simulink model "ExRobotAndEnvironmentControllerContPI"  (Simulink 8.9)
settings: Solver=ode45  StartTime=0.0  StopTime=1000  FixedStep=.01  RelTol=1e-3  EnableMultiTasking=on
values from neighbouring files (symbols this model uses):
  INITIAL_ROBOT_POS_THETA = 1.5    [InitRobotAndEnvironment.m]
  INITIAL_ROBOT_POS_X = 0    [InitRobotAndEnvironment.m]
  INITIAL_ROBOT_POS_Y = 0    [InitRobotAndEnvironment.m]
  INTER_WHEEL_DISTANCE = 0.12    [InitRobotAndEnvironment.m]
  ki_teta = omega*omega/alpha    (= 0.12)    [InitRobotAndEnvironment.m]
  kp_teta = 3*ksi*omega/alpha    (= 0.36)    [InitRobotAndEnvironment.m]
  MAX_SPEED = .5    (= 0.5)    [InitRobotAndEnvironment.m]
  minDistance = 20    [InitRobotAndEnvironment.m]
  ts = SENSOR_SAMPLING_TIME    (= 0.001)    [InitRobotAndEnvironment.m]
  ts_anim = ANIMATION_SAMPLING_TIME    (= 0.01)    [InitRobotAndEnvironment.m]
undefined symbols (not defined in the file or in its folder): Env, Robot, RobotInit
libraries: simulink x3
settings Model: SuppressorTable=22 serialization::archive 11 0 6 0 0 0 11 0  Creator=alex  LastModifiedBy=bonnajul
settings OptimizationCC: ExpressionDepthLimit=2147483647
settings SFSimCC: SimParseCustomCode=off

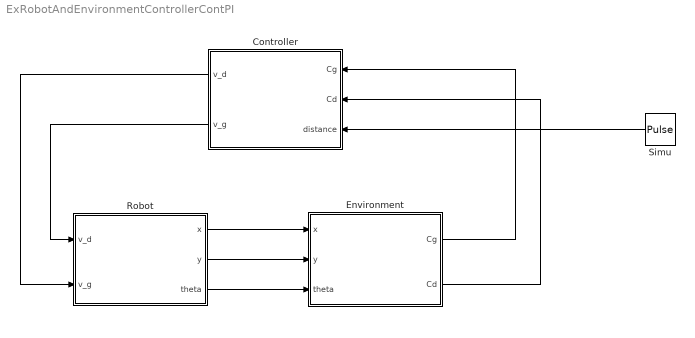
== system ExRobotAndEnvironmentControllerContPI ==
  Controller : Subsystem
  Environment : Subsystem
  Robot : Subsystem
  Simu : DiscretePulseGenerator  PulseType=Time based  Amplitude=25  Period=3  PulseWidth=80
  wires:
  Robot/1(x) -> Environment/1(x)
  Robot/2(y) -> Environment/2(y)
  Robot/3(theta) -> Environment/3(theta)
  Environment/1(Cg) -> Controller/1(Cg)
  Environment/2(Cd) -> Controller/2(Cd)
  Controller/1(v_d) -> Robot/2(v_g)
  Controller/2(v_g) -> Robot/1(v_d)
  Simu/1 -> Controller/3(distance)

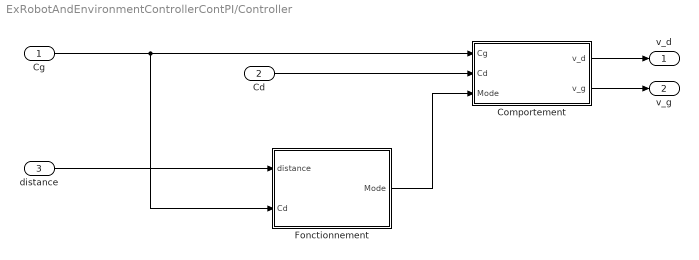
== system ExRobotAndEnvironmentControllerContPI/Controller ==
  Cg : Inport
  Cd : Inport  Port=2
  distance : Inport  Port=3  OutDataTypeStr=double
  Comportement : Subsystem
  Fonctionnement : Subsystem
  v_d : Outport
  v_g : Outport  Port=2
  wires:
  Cg/1 -> Fonctionnement/2("Cd "), Comportement/1(Cg)
  Cd/1 -> Comportement/2(Cd)
  Comportement/1(v_d) -> v_d/1
  Comportement/2(v_g) -> v_g/1
  distance/1 -> Fonctionnement/1(distance)
  Fonctionnement/1(Mode) -> Comportement/3(Mode)

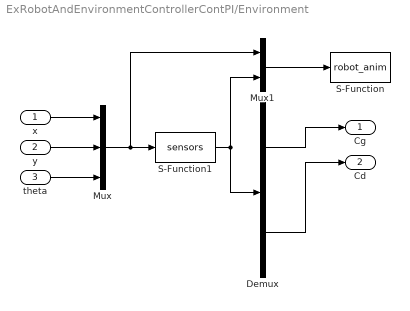
== system ExRobotAndEnvironmentControllerContPI/Environment ==
  x : Inport
  y : Inport  Port=2
  theta : Inport  Port=3
  Demux : Demux  Outputs=2
  Mux : Mux  Inputs=3
  Mux1 : Mux  Inputs=2
  S-Function : S-Function  FunctionName=robot_anim  Parameters=ts_anim,Env,Robot,RobotInit  SFunctionDeploymentMode=off  EnableBusSupport=off
  S-Function1 : S-Function  FunctionName=sensors  Parameters=ts,Env,Robot  SFunctionDeploymentMode=off  EnableBusSupport=off
  Cg : Outport
  Cd : Outport  Port=2
  wires:
  x/1 -> Mux/1
  y/1 -> Mux/2
  theta/1 -> Mux/3
  Mux/1 -> S-Function1/1, Mux1/1
  S-Function1/1 -> Mux1/2, Demux/1
  Mux1/1 -> S-Function/1
  Demux/1 -> Cg/1
  Demux/2 -> Cd/1

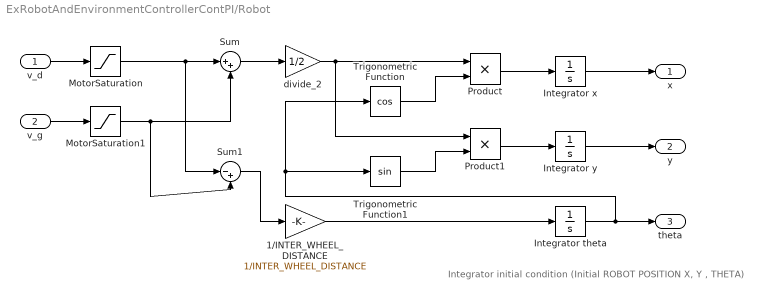
== system ExRobotAndEnvironmentControllerContPI/Robot ==
  note: Integrator initial condition (Initial ROBOT POSITION X, Y , THETA)
  v_d : Inport
  v_g : Inport  Port=2
  1/INTER_WHEEL_DISTANCE : Gain  Gain=1/INTER_WHEEL_DISTANCE
  Integrator theta : Integrator  InitialCondition=INITIAL_ROBOT_POS_THETA
  Integrator x : Integrator  InitialCondition=INITIAL_ROBOT_POS_X
  Integrator y : Integrator  InitialCondition=INITIAL_ROBOT_POS_Y
  MotorSaturation : Saturate  UpperLimit=MAX_SPEED  LowerLimit=-MAX_SPEED
  MotorSaturation1 : Saturate  UpperLimit=MAX_SPEED  LowerLimit=-MAX_SPEED
  Product : Product  RndMeth=Zero
  Product1 : Product  RndMeth=Zero
  Sum : Sum  Inputs=|++
  Sum1 : Sum  Inputs=|-+
  Trigonometric Function : Trigonometry  Operator=cos
  Trigonometric Function1 : Trigonometry
  divide_2 : Gain  Gain=1/2
  x : Outport
  y : Outport  Port=2
  theta : Outport  Port=3
  wires:
  v_d/1 -> MotorSaturation/1
  Integrator x/1 -> x/1
  Integrator y/1 -> y/1
  Integrator theta/1 -> Trigonometric Function/1, Trigonometric Function1/1, theta/1
  Sum/1 -> divide_2/1
  divide_2/1 -> Product1/1, Product/1
  Trigonometric Function/1 -> Product/2
  Trigonometric Function1/1 -> Product1/2
  Product/1 -> Integrator x/1
  Product1/1 -> Integrator y/1
  Sum1/1 -> 1/INTER_WHEEL_DISTANCE/1
  1/INTER_WHEEL_DISTANCE/1 -> Integrator theta/1
  v_g/1 -> MotorSaturation1/1
  MotorSaturation1/1 -> Sum/2, Sum1/2
  MotorSaturation/1 -> Sum/1, Sum1/1

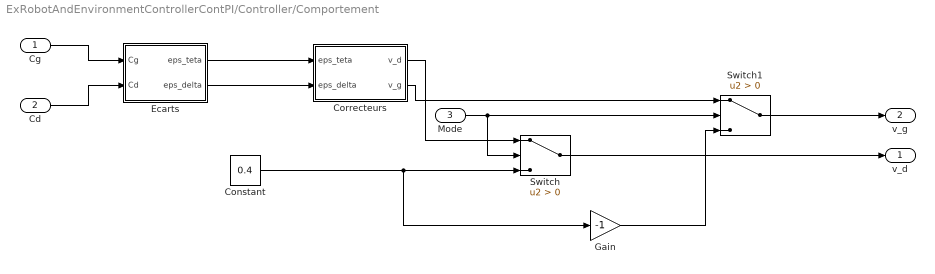
== system ExRobotAndEnvironmentControllerContPI/Controller/Comportement ==
  Cg : Inport  OutDataTypeStr=double
  Cd : Inport  Port=2  OutDataTypeStr=double
  Mode : Inport  Port=3  OutDataTypeStr=boolean
  Constant : Constant  Value=0.4
  "Correcteurs " : Subsystem
  Ecarts : Subsystem
  Gain : Gain  Gain=-1
  Switch : Switch  Criteria=u2 > Threshold
  Switch1 : Switch  Criteria=u2 > Threshold
  v_d : Outport
  v_g : Outport  Port=2
  wires:
  Gain/1 -> Switch1/3
  Mode/1 -> Switch/2, Switch1/2
  Constant/1 -> Gain/1, Switch/3
  "Correcteurs "/1(v_d) -> Switch/1
  Switch1/1 -> v_g/1
  Switch/1 -> v_d/1
  "Correcteurs "/2(v_g) -> Switch1/1
  Ecarts/2(eps_delta) -> "Correcteurs "/2(eps_delta)
  Cd/1 -> Ecarts/2(Cd)
  Cg/1 -> Ecarts/1(Cg)
  Ecarts/1(eps_teta) -> "Correcteurs "/1(eps_teta)

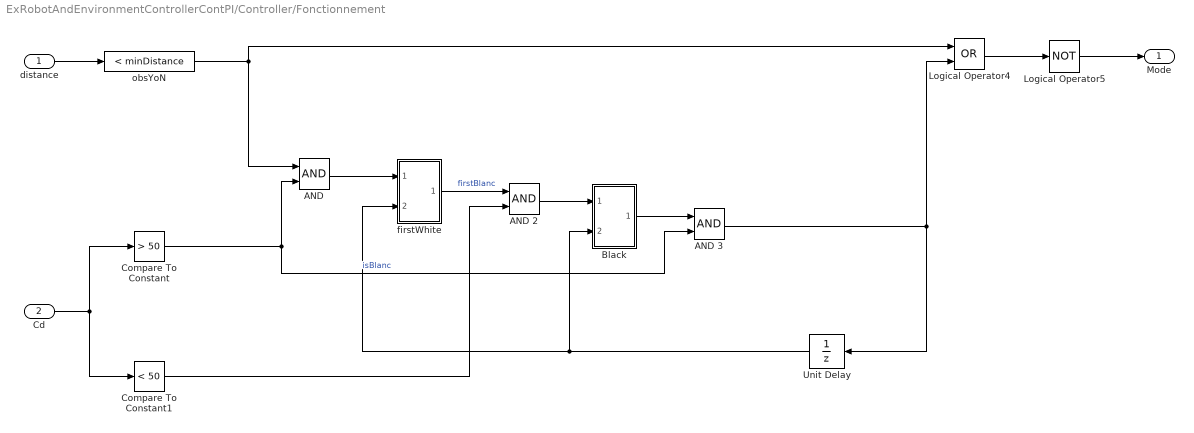
== system ExRobotAndEnvironmentControllerContPI/Controller/Fonctionnement ==
  distance : Inport  OutDataTypeStr=double
  "Cd " : Inport  Port=2  OutDataTypeStr=double
  AND : Logic  AllPortsSameDT=off  OutDataTypeStr=boolean
  AND 2 : Logic  AllPortsSameDT=off  OutDataTypeStr=boolean
  AND 3 : Logic  AllPortsSameDT=off  OutDataTypeStr=boolean
  Black : Subsystem
  Compare To Constant : simulink/Logic and Bit Operations/Compare To Constant  relop=>  const=50  OutDataTypeStr=boolean
  Compare To Constant1 : simulink/Logic and Bit Operations/Compare To Constant  relop=<  const=50  OutDataTypeStr=boolean
  Logical Operator4 : Logic  Operator=OR  AllPortsSameDT=off  OutDataTypeStr=boolean
  Logical Operator5 : Logic  Operator=NOT  AllPortsSameDT=off  OutDataTypeStr=boolean
  Unit Delay : UnitDelay  SampleTime=-1
  "firstWhite " : Subsystem
  obsYoN : simulink/Logic and Bit Operations/Compare To Constant  relop=<  const=minDistance  OutDataTypeStr=boolean
  Mode : Outport
  wires:
  distance/1 -> obsYoN/1
  Compare To Constant/1 -> AND 3/2, AND/2  "isBlanc"
  AND 3/1 -> Unit Delay/1, Logical Operator4/2
  Black/1(Out1) -> AND 3/1
  "firstWhite "/1(Out1) -> AND 2/1  "firstBlanc"
  AND 2/1 -> Black/1(In1)
  obsYoN/1 -> Logical Operator4/1, AND/1
  AND/1 -> "firstWhite "/1(In1)
  Logical Operator4/1 -> Logical Operator5/1
  Unit Delay/1 -> "firstWhite "/2(In2), Black/2(In2)
  Logical Operator5/1 -> Mode/1
  Compare To Constant1/1 -> AND 2/2
  "Cd "/1 -> Compare To Constant1/1, Compare To Constant/1

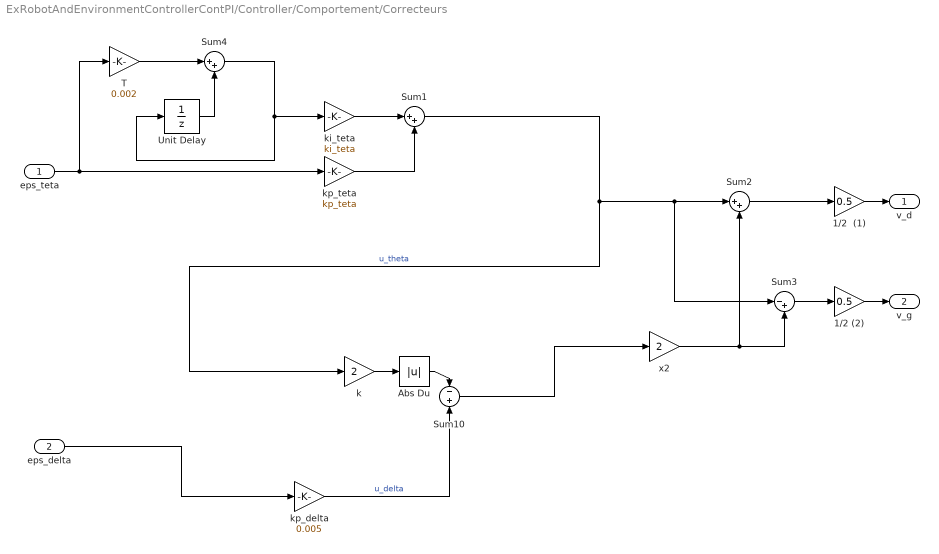
== system ExRobotAndEnvironmentControllerContPI/Controller/Comportement/Correcteurs  ==
  eps_teta : Inport
  eps_delta : Inport  Port=2
  1/2  (1) : Gain  Gain=0.5  SaturateOnIntegerOverflow=on  OutDataTypeStr=Inherit: Same as input  ParamDataTypeStr=Inherit: Same as input
  1/2 (2) : Gain  Gain=0.5  SaturateOnIntegerOverflow=on  OutDataTypeStr=Inherit: Same as input  ParamDataTypeStr=Inherit: Same as input
  Abs Du : Abs  SaturateOnIntegerOverflow=on
  Sum1 : Sum  Inputs=|++  SaturateOnIntegerOverflow=on
  Sum10 : Sum  Inputs=-+  SaturateOnIntegerOverflow=on
  Sum2 : Sum  Inputs=|++  SaturateOnIntegerOverflow=on
  Sum3 : Sum  Inputs=|-+  SaturateOnIntegerOverflow=on
  Sum4 : Sum  Inputs=|++  SaturateOnIntegerOverflow=on
  T : Gain  Gain=0.002  SaturateOnIntegerOverflow=on  OutDataTypeStr=Inherit: Same as input  ParamDataTypeStr=Inherit: Same as input
  Unit Delay : UnitDelay  SampleTime=-1
  k : Gain  Gain=2  SaturateOnIntegerOverflow=on  OutDataTypeStr=Inherit: Same as input  ParamDataTypeStr=Inherit: Same as input
  ki_teta : Gain  Gain=ki_teta  SaturateOnIntegerOverflow=on  OutDataTypeStr=Inherit: Same as input  ParamDataTypeStr=Inherit: Same as input
  kp_delta : Gain  Gain=0.005
  kp_teta : Gain  Gain=kp_teta  SaturateOnIntegerOverflow=on  OutDataTypeStr=Inherit: Same as input  ParamDataTypeStr=Inherit: Same as input
  x2 : Gain  Gain=2  SaturateOnIntegerOverflow=on  OutDataTypeStr=Inherit: Same as input  ParamDataTypeStr=Inherit: Same as input
  v_d : Outport
  v_g : Outport  Port=2
  wires:
  ki_teta/1 -> Sum1/1
  kp_teta/1 -> Sum1/2
  Sum2/1 -> 1/2  (1)/1
  Sum3/1 -> 1/2 (2)/1
  k/1 -> Abs Du/1
  kp_delta/1 -> Sum10/2  "u_delta"
  eps_teta/1 -> T/1, kp_teta/1
  Abs Du/1 -> Sum10/1
  x2/1 -> Sum2/2, Sum3/2
  Sum10/1 -> x2/1
  Sum1/1 -> k/1, Sum2/1, Sum3/1  "u_theta"
  1/2  (1)/1 -> v_d/1
  1/2 (2)/1 -> v_g/1
  eps_delta/1 -> kp_delta/1
  T/1 -> Sum4/1
  Unit Delay/1 -> Sum4/2
  Sum4/1 -> Unit Delay/1, ki_teta/1

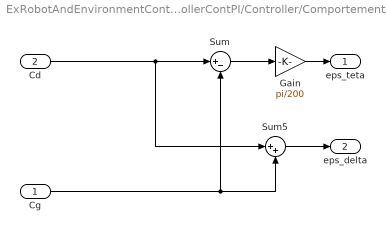
== system ExRobotAndEnvironmentControllerContPI/Controller/Comportement/Ecarts ==
  Cg : Inport
  Cd : Inport  Port=2
  Gain : Gain  Gain=pi/200
  Sum : Sum  Inputs=|+-
  Sum5 : Sum  Inputs=|++
  eps_teta : Outport
  eps_delta : Outport  Port=2
  wires:
  Sum/1 -> Gain/1
  Cd/1 -> Sum/1, Sum5/1
  Cg/1 -> Sum/2, Sum5/2
  Gain/1 -> eps_teta/1
  Sum5/1 -> eps_delta/1

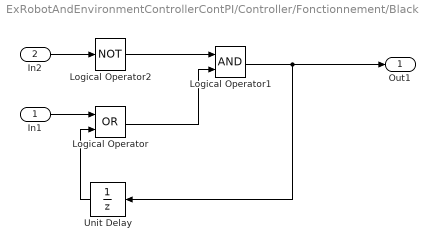
== system ExRobotAndEnvironmentControllerContPI/Controller/Fonctionnement/Black ==
  In1 : Inport
  In2 : Inport  Port=2
  Logical Operator : Logic  Operator=OR  AllPortsSameDT=off  OutDataTypeStr=boolean
  Logical Operator1 : Logic  AllPortsSameDT=off  OutDataTypeStr=boolean
  Logical Operator2 : Logic  Operator=NOT  AllPortsSameDT=off  OutDataTypeStr=boolean
  Unit Delay : UnitDelay  SampleTime=-1
  Out1 : Outport
  wires:
  In1/1 -> Logical Operator/1
  Unit Delay/1 -> Logical Operator/2
  Logical Operator/1 -> Logical Operator1/2
  In2/1 -> Logical Operator2/1
  Logical Operator1/1 -> Out1/1, Unit Delay/1
  Logical Operator2/1 -> Logical Operator1/1

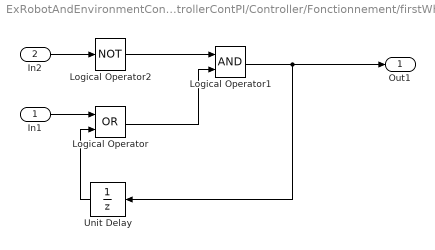
== system ExRobotAndEnvironmentControllerContPI/Controller/Fonctionnement/firstWhite  ==
  In1 : Inport
  In2 : Inport  Port=2
  Logical Operator : Logic  Operator=OR  AllPortsSameDT=off  OutDataTypeStr=boolean
  Logical Operator1 : Logic  AllPortsSameDT=off  OutDataTypeStr=boolean
  Logical Operator2 : Logic  Operator=NOT  AllPortsSameDT=off  OutDataTypeStr=boolean
  Unit Delay : UnitDelay  SampleTime=-1
  Out1 : Outport
  wires:
  In1/1 -> Logical Operator/1
  Unit Delay/1 -> Logical Operator/2
  Logical Operator/1 -> Logical Operator1/2
  In2/1 -> Logical Operator2/1
  Logical Operator1/1 -> Out1/1, Unit Delay/1
  Logical Operator2/1 -> Logical Operator1/1
